simulink model "cruiseControl"  (R2023a)
settings: Solver=VariableStepAuto  StartTime=0.0  StopTime=120  RelTol=1e-3
values from neighbouring files (symbols this model uses):
  b = 50    [PIcontrol.m]    (also in cruiseControl.m; linearModelSim.m)
  m = 1000    [PIcontrol.m]    (also in cruiseControl.m; linearModelSim.m)
settings Model: Creator=shrey  LastModifiedBy=shrey

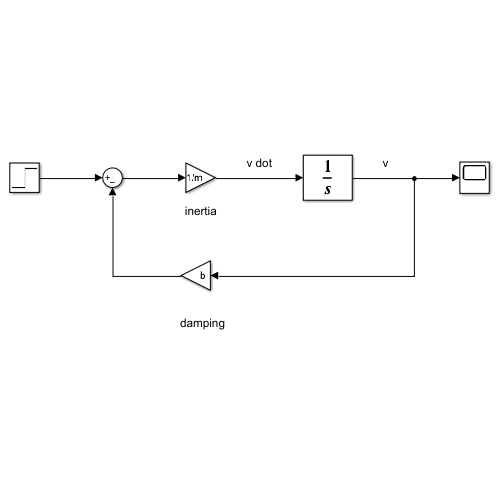
[thumbnail: Simulink's stored preview of the top-level diagram]
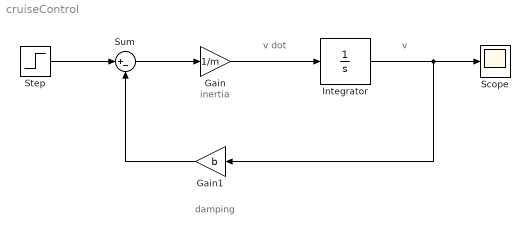
== system cruiseControl ==
  note: v dot
  note: v
  note: inertia
  note: damping
  Gain : Gain  Gain=1/m
  Gain1 : Gain  Gain=b
  Integrator : Integrator
  Scope : Scope
  Step : Step  Time=0  After=u  SampleTime=0
  Sum : Sum  Inputs=|+-
  wires:
  Gain/1 -> Integrator/1
  Integrator/1 -> Scope/1, Gain1/1
  Sum/1 -> Gain/1
  Gain1/1 -> Sum/2
  Step/1 -> Sum/1
